simulink model "PhaseToTimeRefMod empty"  (R2016b)
settings: Solver=VariableStepAuto  StartTime=0.0  StopTime=10.0  RelTol=1e-3
settings Model: DataDictionary=DataDictionary.sldd  Creator=lucadelaat  LastModifiedBy=Taeke

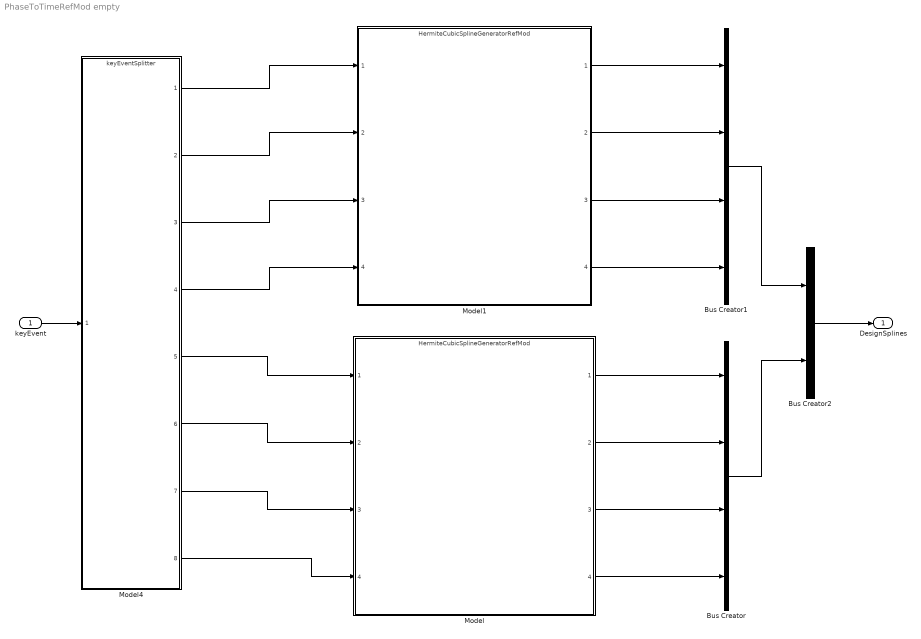
== system PhaseToTimeRefMod empty ==
  keyEvent : Inport  OutDataTypeStr=Bus: keyEventTotal  BusOutputAsStruct=on
  Bus Creator : BusCreator  Inputs=4
  Bus Creator1 : BusCreator  Inputs=4
  Bus Creator2 : BusCreator  Inputs=2
  Model : ModelReference  ModelNameDialog=HermiteCubicSplineGeneratorRefMod.slx  SimulationMode=Normal  ModelReferenceVersion=1.17
  Model1 : ModelReference  ModelNameDialog=HermiteCubicSplineGeneratorRefMod.slx  SimulationMode=Normal  ModelReferenceVersion=1.17
  Model4 : ModelReference  ModelNameDialog=keyEventSplitter.slx  SimulationMode=Normal  ModelReferenceVersion=1.3
  DesignSplines : Outport  OutDataTypeStr=Bus: designSplineTotal
  wires:
  Model4/3 -> Model1/3
  Model4/4 -> Model1/4
  Model4/6 -> Model/2
  Model4/7 -> Model/3
  Model4/8 -> Model/4
  Model4/2 -> Model1/2
  Model4/1 -> Model1/1
  Model4/5 -> Model/1
  keyEvent/1 -> Model4/1
  Model/1 -> Bus Creator/1
  Model/4 -> Bus Creator/4
  Model/3 -> Bus Creator/3
  Model/2 -> Bus Creator/2
  Model1/1 -> Bus Creator1/1
  Model1/3 -> Bus Creator1/3
  Model1/4 -> Bus Creator1/4
  Model1/2 -> Bus Creator1/2
  Bus Creator1/1 -> Bus Creator2/1
  Bus Creator/1 -> Bus Creator2/2
  Bus Creator2/1 -> DesignSplines/1
